simulink model "MotorController_PID_Simulink"  (R2020a)
settings: Solver=VariableStepAuto  StartTime=0.0  StopTime=10.0  RelTol=1e-3
settings Model: Creator=Oguzhan  LastModifiedBy=oguzhan
settings DataIOCC: ReturnWorkspaceOutputs=off
settings DebuggingCC: ArithmeticOperatorsInVariantConditions=warning
settings SFSimCC: SimUseLocalCustomCode=off  CustomCodeUndefinedFunction=UseInterfaceOnly
settings RTWCC: RTWUseLocalCustomCode=off

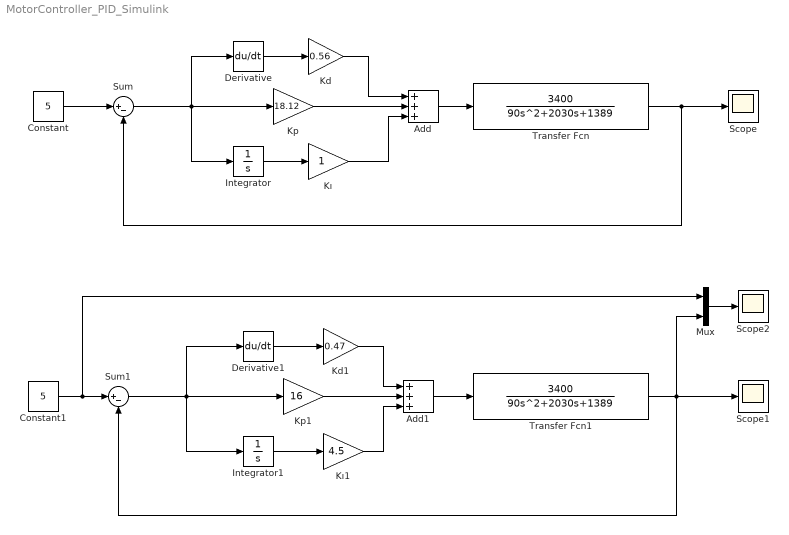
== system MotorController_PID_Simulink ==
  Add : Sum  Inputs=+++
  Add1 : Sum  Inputs=+++
  Constant : Constant  Value=5
  Constant1 : Constant  Value=5
  Derivative : Derivative
  Derivative1 : Derivative
  Integrator : Integrator
  Integrator1 : Integrator
  Kd : Gain  Gain=0.56
  Kd1 : Gain  Gain=0.47
  Kp : Gain  Gain=18.12
  Kp1 : Gain  Gain=16
  "Kı " : Gain
  Kı1 : Gain  Gain=4.5
  Mux : Mux  Inputs=2
  Scope : Scope
  Scope1 : Scope
  Scope2 : Scope
  Sum : Sum  Inputs=|+-
  Sum1 : Sum  Inputs=|+-
  Transfer Fcn : TransferFcn  Numerator=[3400]  Denominator=[90 2030 1389]
  Transfer Fcn1 : TransferFcn  Numerator=[3400]  Denominator=[90 2030 1389]
  wires:
  Transfer Fcn/1 -> Sum/2, Scope/1
  Constant/1 -> Sum/1
  Add/1 -> Transfer Fcn/1
  Kp/1 -> Add/2
  Sum/1 -> Derivative/1, Integrator/1, Kp/1
  Derivative/1 -> Kd/1
  Kd/1 -> Add/1
  Integrator/1 -> "Kı "/1
  "Kı "/1 -> Add/3
  Kı1/1 -> Add1/3
  Integrator1/1 -> Kı1/1
  Constant1/1 -> Mux/1, Sum1/1
  Kd1/1 -> Add1/1
  Kp1/1 -> Add1/2
  Sum1/1 -> Derivative1/1, Integrator1/1, Kp1/1
  Transfer Fcn1/1 -> Mux/2, Sum1/2, Scope1/1
  Add1/1 -> Transfer Fcn1/1
  Derivative1/1 -> Kd1/1
  Mux/1 -> Scope2/1
